simulink subsystem "controller_subsystem"  (R2025b)
settings: Solver=VariableStepAuto  StartTime=0.0  StopTime=10.0  RelTol=1e-3
settings Model: Creator=sanborkl  LastModifiedBy=sanborkl

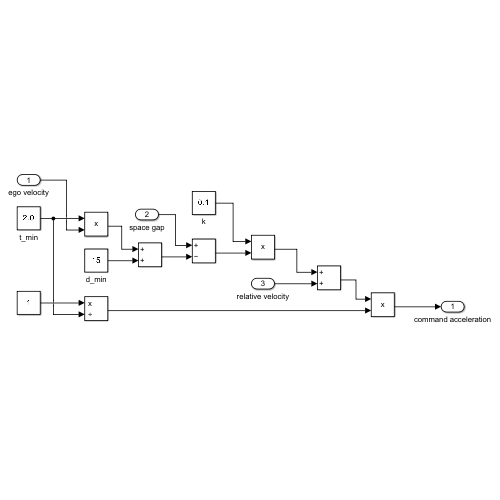
[thumbnail: Simulink's stored preview of the top-level diagram]
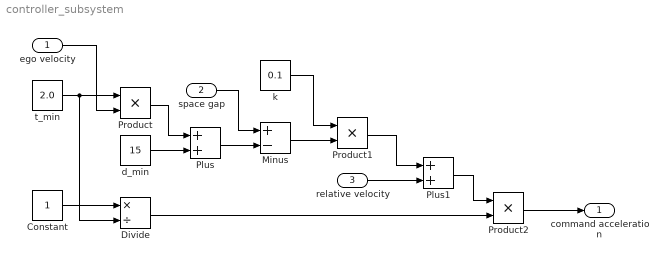
== system controller_subsystem ==
  ego velocity : Inport
  space gap : Inport  Port=2
  relative velocity : Inport  Port=3
  Constant : Constant
  Divide : Product  Inputs=*/
  Minus : Sum  Inputs=+-
  Plus : Sum
  Plus1 : Sum
  Product : Product
  Product1 : Product
  Product2 : Product
  d_min : Constant  Value=15
  k : Constant  Value=0.1
  t_min : Constant  Value=2.0
  command acceleration : Outport
  wires:
  ego velocity/1 -> Product/2
  t_min/1 -> Divide/2, Product/1
  d_min/1 -> Plus/2
  Constant/1 -> Divide/1
  Product/1 -> Plus/1
  Divide/1 -> Product2/2
  relative velocity/1 -> Plus1/2
  space gap/1 -> Minus/1
  Plus/1 -> Minus/2
  k/1 -> Product1/1
  Minus/1 -> Product1/2
  Product1/1 -> Plus1/1
  Plus1/1 -> Product2/1
  Product2/1 -> command acceleration/1
